simulink model "helix_drone_competition"  (R2022b)
settings: Solver=VariableStepAuto  StartTime=0.0  StopTime=10.0  RelTol=1e-3
settings Model: Creator=gerve  LastModifiedBy=gerve

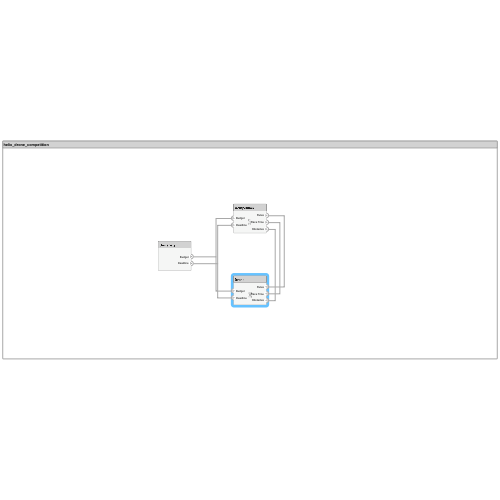
[thumbnail: Simulink's stored preview of the top-level diagram]
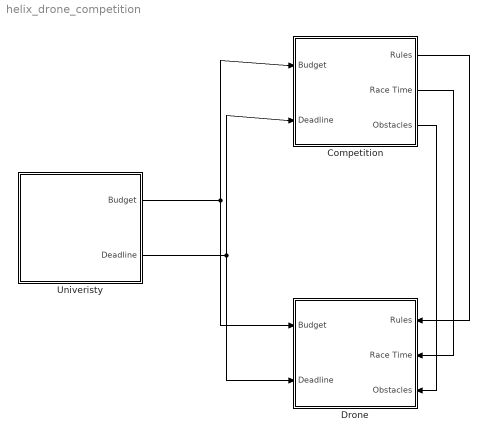
== system helix_drone_competition ==
  Competition : Subsystem
      settings: PortSchema="{\"entries\":[{\"content\":{\"headerSize\":26,\"margin\":15,\"minimumSpacing\":25,\"sides\":[{\"content\":{\"connectorIds\":[\"In1\",\"In2\"]},\"type\":\"ConnectorPlacement.EquallySpacedRectSide\",\"uuid\":\"f32b2b14-41b4-41d2-98c7-b99e10502cf5\"},{\"content\":{\"connectorIds\":[\"Out1\",\"Out2\",\"Out3\"],\"side\":\"RIGHT\"},\"type\":\"ConnectorPlacement.EquallySpacedRectSide\",\"uuid\":\"ebd87c84-7864-4900-8797-b3d9295a8a40\"},{\"content\":{\"connectorIds\":[],\"side\":\"TOP\"},\"type\":\"ConnectorPlacement.EquallySpacedRectSide\",\"uuid\":\"98bce1a8-04c7-44b4-bd36-c653bce1592e\"}]},\"type\":\"ConnectorPlacement.EquallySpacedConnector\",\"uuid\":\"4aeaf037-8c3a-4b17-97e2-80e7a9f8e112\"}],\"packageUris\":[\"http://schema.mathworks.com/mf0/Connector/R2020b\"],\"version\":\"1.0\"}"
  Drone : Subsystem  RequirementInfo="{}  %GIDa_630028c7_c920_43e1_b933_7776371f28a3"
      settings: PortSchema="{\"entries\":[{\"content\":{\"headerSize\":26,\"margin\":15,\"minimumSpacing\":25,\"sides\":[{\"content\":{\"connectorIds\":[\"In4\",\"In5\"]},\"type\":\"ConnectorPlacement.EquallySpacedRectSide\",\"uuid\":\"f32b2b14-41b4-41d2-98c7-b99e10502cf5\"},{\"content\":{\"connectorIds\":[\"In1\",\"In2\",\"In3\"],\"side\":\"RIGHT\"},\"type\":\"ConnectorPlacement.EquallySpacedRectSide\",\"uuid\":\"ebd87c84-7864-4900-8797-b3d9295a8a40\"},{\"content\":{\"connectorIds\":[],\"side\":\"TOP\"},\"type\":\"ConnectorPlacement.EquallySpacedRectSide\",\"uuid\":\"98bce1a8-04c7-44b4-bd36-c653bce1592e\"}]},\"type\":\"ConnectorPlacement.EquallySpacedConnector\",\"uuid\":\"4aeaf037-8c3a-4b17-97e2-80e7a9f8e112\"}],\"packageUris\":[\"http://schema.mathworks.com/mf0/Connector/R2020b\"],\"version\":\"1.0\"}"
  Univeristy : Subsystem
      settings: PortSchema="{\"entries\":[{\"content\":{\"headerSize\":26,\"margin\":15,\"minimumSpacing\":25,\"sides\":[{\"content\":{\"connectorIds\":[]},\"type\":\"ConnectorPlacement.EquallySpacedRectSide\",\"uuid\":\"f32b2b14-41b4-41d2-98c7-b99e10502cf5\"},{\"content\":{\"connectorIds\":[\"Out1\",\"Out2\"],\"side\":\"RIGHT\"},\"type\":\"ConnectorPlacement.EquallySpacedRectSide\",\"uuid\":\"ebd87c84-7864-4900-8797-b3d9295a8a40\"},{\"content\":{\"connectorIds\":[],\"side\":\"TOP\"},\"type\":\"ConnectorPlacement.EquallySpacedRectSide\",\"uuid\":\"98bce1a8-04c7-44b4-bd36-c653bce1592e\"}]},\"type\":\"ConnectorPlacement.EquallySpacedConnector\",\"uuid\":\"4aeaf037-8c3a-4b17-97e2-80e7a9f8e112\"}],\"packageUris\":[\"http://schema.mathworks.com/mf0/Connector/R2020b\"],\"version\":\"1.0\"}"
  wires:
  Univeristy/1(Budget) -> Competition/1(Budget), Drone/4(Budget)
  Univeristy/2(Deadline) -> Competition/2(Deadline), Drone/5(Deadline)
  Competition/1(Rules) -> Drone/1(Rules)
  Competition/2(Race Time) -> Drone/2(Race Time)
  Competition/3(Obstacles) -> Drone/3(Obstacles)

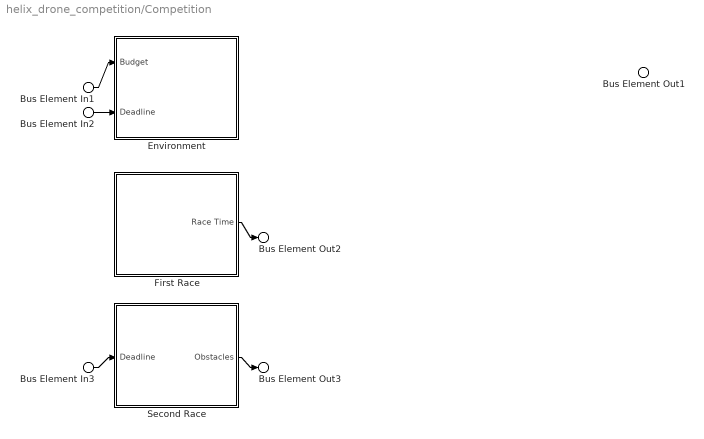
== system helix_drone_competition/Competition ==
  Bus Element In1 : Inport  PortName=Budget
  Bus Element In3 : Inport  PortName=Budget
  Bus Element In2 : Inport  Port=2  PortName=Deadline
  Environment : Subsystem
      settings: PortSchema="{\"entries\":[{\"content\":{\"headerSize\":26,\"margin\":15,\"minimumSpacing\":25,\"sides\":[{\"content\":{\"connectorIds\":[\"In1\",\"In2\"]},\"type\":\"ConnectorPlacement.EquallySpacedRectSide\",\"uuid\":\"f32b2b14-41b4-41d2-98c7-b99e10502cf5\"},{\"content\":{\"connectorIds\":[],\"side\":\"RIGHT\"},\"type\":\"ConnectorPlacement.EquallySpacedRectSide\",\"uuid\":\"ebd87c84-7864-4900-8797-b3d9295a8a40\"},{\"content\":{\"connectorIds\":[],\"side\":\"TOP\"},\"type\":\"ConnectorPlacement.EquallySpacedRectSide\",\"uuid\":\"98bce1a8-04c7-44b4-bd36-c653bce1592e\"}]},\"type\":\"ConnectorPlacement.EquallySpacedConnector\",\"uuid\":\"4aeaf037-8c3a-4b17-97e2-80e7a9f8e112\"}],\"packageUris\":[\"http://schema.mathworks.com/mf0/Connector/R2020b\"],\"version\":\"1.0\"}"
  First Race : Subsystem
      settings: PortSchema="{\"entries\":[{\"content\":{\"headerSize\":26,\"margin\":15,\"minimumSpacing\":25,\"sides\":[{\"content\":{\"connectorIds\":[]},\"type\":\"ConnectorPlacement.EquallySpacedRectSide\",\"uuid\":\"f32b2b14-41b4-41d2-98c7-b99e10502cf5\"},{\"content\":{\"connectorIds\":[\"Out1\"],\"side\":\"RIGHT\"},\"type\":\"ConnectorPlacement.EquallySpacedRectSide\",\"uuid\":\"ebd87c84-7864-4900-8797-b3d9295a8a40\"},{\"content\":{\"connectorIds\":[],\"side\":\"TOP\"},\"type\":\"ConnectorPlacement.EquallySpacedRectSide\",\"uuid\":\"98bce1a8-04c7-44b4-bd36-c653bce1592e\"}]},\"type\":\"ConnectorPlacement.EquallySpacedConnector\",\"uuid\":\"4aeaf037-8c3a-4b17-97e2-80e7a9f8e112\"}],\"packageUris\":[\"http://schema.mathworks.com/mf0/Connector/R2020b\"],\"version\":\"1.0\"}"
  Second Race : Subsystem
      settings: PortSchema="{\"entries\":[{\"content\":{\"headerSize\":26,\"margin\":15,\"minimumSpacing\":25,\"sides\":[{\"content\":{\"connectorIds\":[\"In1\"]},\"type\":\"ConnectorPlacement.EquallySpacedRectSide\",\"uuid\":\"f32b2b14-41b4-41d2-98c7-b99e10502cf5\"},{\"content\":{\"connectorIds\":[\"Out1\"],\"side\":\"RIGHT\"},\"type\":\"ConnectorPlacement.EquallySpacedRectSide\",\"uuid\":\"ebd87c84-7864-4900-8797-b3d9295a8a40\"},{\"content\":{\"connectorIds\":[],\"side\":\"TOP\"},\"type\":\"ConnectorPlacement.EquallySpacedRectSide\",\"uuid\":\"98bce1a8-04c7-44b4-bd36-c653bce1592e\"}]},\"type\":\"ConnectorPlacement.EquallySpacedConnector\",\"uuid\":\"4aeaf037-8c3a-4b17-97e2-80e7a9f8e112\"}],\"packageUris\":[\"http://schema.mathworks.com/mf0/Connector/R2020b\"],\"version\":\"1.0\"}"
  Bus Element Out1 : Outport  PortName=Rules
  Bus Element Out2 : Outport  Port=2  PortName=Race Time
  Bus Element Out3 : Outport  Port=3  PortName=Obstacles
  wires:
  Bus Element In1/1 -> Environment/1(Budget)
  Second Race/1(Obstacles) -> Bus Element Out3/1
  First Race/1(Race Time) -> Bus Element Out2/1
  Bus Element In3/1 -> Second Race/1(Deadline)
  Bus Element In2/1 -> Environment/2(Deadline)

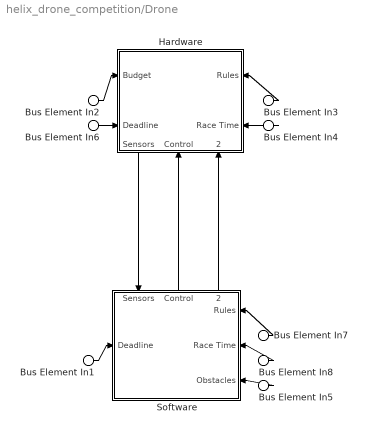
== system helix_drone_competition/Drone ==
  Bus Element In3 : Inport  PortName=Rules
  Bus Element In7 : Inport  PortName=Rules
  Bus Element In4 : Inport  Port=2  PortName=Race Time
  Bus Element In8 : Inport  Port=2  PortName=Race Time
  Bus Element In5 : Inport  Port=3  PortName=Obstacles
  Bus Element In2 : Inport  Port=4  PortName=Budget
  Bus Element In1 : Inport  Port=5  PortName=Deadline
  Bus Element In6 : Inport  Port=5  PortName=Deadline
  Hardware : Subsystem
      settings: PortSchema="{\"entries\":[{\"content\":{\"headerSize\":26,\"margin\":15,\"minimumSpacing\":25,\"sides\":[{\"content\":{\"connectorIds\":[\"In5\",\"In6\"]},\"type\":\"ConnectorPlacement.EquallySpacedRectSide\",\"uuid\":\"f32b2b14-41b4-41d2-98c7-b99e10502cf5\"},{\"content\":{\"connectorIds\":[\"In3\",\"In4\"],\"side\":\"RIGHT\"},\"type\":\"ConnectorPlacement.EquallySpacedRectSide\",\"uuid\":\"ebd87c84-7864-4900-8797-b3d9295a8a40\"},{\"content\":{\"connectorIds\":[],\"side\":\"TOP\"},\"type\":\"ConnectorPlacement.EquallySpacedRectSide\",\"uuid\":\"98bce1a8-04c7-44b4-bd36-c653bce1592e\"},{\"content\":{\"connectorIds\":[\"Out1\",\"In1\",\"In2\"],\"side\":\"BOTTOM\"},\"type\":\"ConnectorPlacement.EquallySpacedRectSide\",\"uuid\":\"b8bbf94b-b15d-45e5-9284-c94e35cda025\"}]},\"type\":\"ConnectorPlacement.EquallySpacedConnector\",\"uuid\":\"4aeaf037-8c3a-4b17-97e2-80e7a9f8e112\"}],\"packageUris\":[\"http://schema.mathworks.com/mf0/Connector/R2020b\"],\"version\":\"1.0\"}"
  Software : Subsystem
      settings: PortSchema="{\"entries\":[{\"content\":{\"headerSize\":26,\"margin\":15,\"minimumSpacing\":25,\"sides\":[{\"content\":{\"connectorIds\":[\"In5\"]},\"type\":\"ConnectorPlacement.EquallySpacedRectSide\",\"uuid\":\"f32b2b14-41b4-41d2-98c7-b99e10502cf5\"},{\"content\":{\"connectorIds\":[\"In2\",\"In3\",\"In4\"],\"side\":\"RIGHT\"},\"type\":\"ConnectorPlacement.EquallySpacedRectSide\",\"uuid\":\"ebd87c84-7864-4900-8797-b3d9295a8a40\"},{\"content\":{\"connectorIds\":[\"In1\",\"Out1\",\"Out2\"],\"side\":\"TOP\"},\"type\":\"ConnectorPlacement.EquallySpacedRectSide\",\"uuid\":\"98bce1a8-04c7-44b4-bd36-c653bce1592e\"},{\"content\":{\"connectorIds\":[],\"side\":\"BOTTOM\"},\"type\":\"ConnectorPlacement.EquallySpacedRectSide\",\"uuid\":\"176a6af5-98df-42e2-83ff-7372f5d8c599\"}]},\"type\":\"ConnectorPlacement.EquallySpacedConnector\",\"uuid\":\"4aeaf037-8c3a-4b17-97e2-80e7a9f8e112\"}],\"packageUris\":[\"http://schema.mathworks.com/mf0/Connector/R2020b\"],\"version\":\"1.0\"}"
  wires:
  Bus Element In2/1 -> Hardware/5(Budget)
  Bus Element In1/1 -> Software/5(Deadline)
  Bus Element In6/1 -> Hardware/6(Deadline)
  Bus Element In3/1 -> Hardware/3(Rules)
  Bus Element In7/1 -> Software/2(Rules)
  Bus Element In4/1 -> Hardware/4(Race Time)
  Bus Element In8/1 -> Software/3(Race Time)
  Bus Element In5/1 -> Software/4(Obstacles)
  Software/2(Instructions) -> Hardware/2(Instructions)
  Hardware/1(Sensors) -> Software/1(Sensors)
  Software/1(Control) -> Hardware/1(Control)

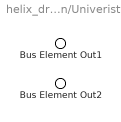
== system helix_drone_competition/Univeristy ==
  Bus Element Out1 : Outport  PortName=Budget
  Bus Element Out2 : Outport  Port=2  PortName=Deadline

== system helix_drone_competition/Competition/Environment ==
  Bus Element In1 : Inport  PortName=Budget
  Bus Element In2 : Inport  Port=2  PortName=Deadline

== system helix_drone_competition/Competition/First Race ==
  Bus Element Out1 : Outport  PortName=Race Time

== system helix_drone_competition/Competition/Second Race ==
  Bus Element In1 : Inport  PortName=Deadline
  Bus Element Out1 : Outport  PortName=Obstacles

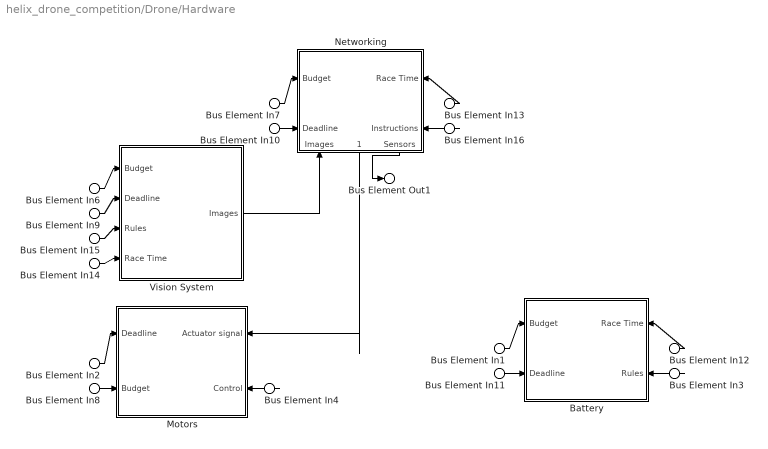
== system helix_drone_competition/Drone/Hardware ==
  Bus Element In4 : Inport  PortName=Control
  Bus Element In16 : Inport  Port=2  PortName=Instructions
  Bus Element In3 : Inport  Port=3  PortName=Rules
  Bus Element In15 : Inport  Port=3  PortName=Rules
  Bus Element In12 : Inport  Port=4  PortName=Race Time
  Bus Element In13 : Inport  Port=4  PortName=Race Time
  Bus Element In14 : Inport  Port=4  PortName=Race Time
  Bus Element In{1,6..8} (4 alike) : Inport  Port=5  PortName=Budget
  Bus Element In{2,9..11} (4 alike) : Inport  Port=6  PortName=Deadline
  Battery : Subsystem
      settings: PortSchema="{\"entries\":[{\"content\":{\"headerSize\":26,\"margin\":15,\"minimumSpacing\":25,\"sides\":[{\"content\":{\"connectorIds\":[\"In3\",\"In4\"]},\"type\":\"ConnectorPlacement.EquallySpacedRectSide\",\"uuid\":\"f32b2b14-41b4-41d2-98c7-b99e10502cf5\"},{\"content\":{\"connectorIds\":[\"In1\",\"In2\"],\"side\":\"RIGHT\"},\"type\":\"ConnectorPlacement.EquallySpacedRectSide\",\"uuid\":\"ebd87c84-7864-4900-8797-b3d9295a8a40\"},{\"content\":{\"connectorIds\":[],\"side\":\"TOP\"},\"type\":\"ConnectorPlacement.EquallySpacedRectSide\",\"uuid\":\"98bce1a8-04c7-44b4-bd36-c653bce1592e\"}]},\"type\":\"ConnectorPlacement.EquallySpacedConnector\",\"uuid\":\"4aeaf037-8c3a-4b17-97e2-80e7a9f8e112\"}],\"packageUris\":[\"http://schema.mathworks.com/mf0/Connector/R2020b\"],\"version\":\"1.0\"}"
  Motors : Subsystem
      settings: PortSchema="{\"entries\":[{\"content\":{\"headerSize\":26,\"margin\":15,\"minimumSpacing\":25,\"sides\":[{\"content\":{\"connectorIds\":[\"In3\",\"In4\"]},\"type\":\"ConnectorPlacement.EquallySpacedRectSide\",\"uuid\":\"f32b2b14-41b4-41d2-98c7-b99e10502cf5\"},{\"content\":{\"connectorIds\":[\"In1\",\"In2\"],\"side\":\"RIGHT\"},\"type\":\"ConnectorPlacement.EquallySpacedRectSide\",\"uuid\":\"ebd87c84-7864-4900-8797-b3d9295a8a40\"},{\"content\":{\"connectorIds\":[],\"side\":\"TOP\"},\"type\":\"ConnectorPlacement.EquallySpacedRectSide\",\"uuid\":\"98bce1a8-04c7-44b4-bd36-c653bce1592e\"}]},\"type\":\"ConnectorPlacement.EquallySpacedConnector\",\"uuid\":\"4aeaf037-8c3a-4b17-97e2-80e7a9f8e112\"}],\"packageUris\":[\"http://schema.mathworks.com/mf0/Connector/R2020b\"],\"version\":\"1.0\"}"
  Networking : Subsystem
      settings: PortSchema="{\"entries\":[{\"content\":{\"headerSize\":26,\"margin\":15,\"minimumSpacing\":25,\"sides\":[{\"content\":{\"connectorIds\":[\"In4\",\"In5\"]},\"type\":\"ConnectorPlacement.EquallySpacedRectSide\",\"uuid\":\"f32b2b14-41b4-41d2-98c7-b99e10502cf5\"},{\"content\":{\"connectorIds\":[\"In2\",\"In3\"],\"side\":\"RIGHT\"},\"type\":\"ConnectorPlacement.EquallySpacedRectSide\",\"uuid\":\"ebd87c84-7864-4900-8797-b3d9295a8a40\"},{\"content\":{\"connectorIds\":[],\"side\":\"TOP\"},\"type\":\"ConnectorPlacement.EquallySpacedRectSide\",\"uuid\":\"98bce1a8-04c7-44b4-bd36-c653bce1592e\"},{\"content\":{\"connectorIds\":[\"In1\",\"Out1\",\"Out2\"],\"side\":\"BOTTOM\"},\"type\":\"ConnectorPlacement.EquallySpacedRectSide\",\"uuid\":\"347c56eb-8d07-4315-bae9-6dad91ea2500\"}]},\"type\":\"ConnectorPlacement.EquallySpacedConnector\",\"uuid\":\"4aeaf037-8c3a-4b17-97e2-80e7a9f8e112\"}],\"packageUris\":[\"http://schema.mathworks.com/mf0/Connector/R2020b\"],\"version\":\"1.0\"}"
  Vision System : Subsystem
      settings: PortSchema="{\"entries\":[{\"content\":{\"headerSize\":26,\"margin\":15,\"minimumSpacing\":25,\"sides\":[{\"content\":{\"connectorIds\":[\"In3\",\"In4\",\"In2\",\"In1\"]},\"type\":\"ConnectorPlacement.EquallySpacedRectSide\",\"uuid\":\"f32b2b14-41b4-41d2-98c7-b99e10502cf5\"},{\"content\":{\"connectorIds\":[\"Out1\"],\"side\":\"RIGHT\"},\"type\":\"ConnectorPlacement.EquallySpacedRectSide\",\"uuid\":\"ebd87c84-7864-4900-8797-b3d9295a8a40\"},{\"content\":{\"connectorIds\":[],\"side\":\"TOP\"},\"type\":\"ConnectorPlacement.EquallySpacedRectSide\",\"uuid\":\"98bce1a8-04c7-44b4-bd36-c653bce1592e\"},{\"content\":{\"connectorIds\":[],\"side\":\"BOTTOM\"},\"type\":\"ConnectorPlacement.EquallySpacedRectSide\",\"uuid\":\"726fdaec-6ead-4202-81de-1add9a01df27\"}]},\"type\":\"ConnectorPlacement.EquallySpacedConnector\",\"uuid\":\"4aeaf037-8c3a-4b17-97e2-80e7a9f8e112\"}],\"packageUris\":[\"http://schema.mathworks.com/mf0/Connector/R2020b\"],\"version\":\"1.0\"}"
  Bus Element Out1 : Outport  PortName=Sensors
  wires:
  Bus Element In9/1 -> Vision System/4(Deadline)
  Bus Element In10/1 -> Networking/5(Deadline)
  Bus Element In11/1 -> Battery/4(Deadline)
  Bus Element In1/1 -> Battery/3(Budget)
  Bus Element In6/1 -> Vision System/3(Budget)
  Bus Element In15/1 -> Vision System/2(Rules)
  Bus Element In14/1 -> Vision System/1(Race Time)
  Bus Element In8/1 -> Motors/4(Budget)
  Bus Element In7/1 -> Networking/4(Budget)
  Vision System/1(Images) -> Networking/1(Images)
  Networking/2(Sensors) -> Bus Element Out1/1
  Networking/1(Actuator signal) -> Motors/1(Actuator signal)
  Bus Element In13/1 -> Networking/2(Race Time)
  Bus Element In12/1 -> Battery/1(Race Time)
  Bus Element In3/1 -> Battery/2(Rules)
  Bus Element In2/1 -> Motors/3(Deadline)
  Bus Element In16/1 -> Networking/3(Instructions)
  Bus Element In4/1 -> Motors/2(Control)

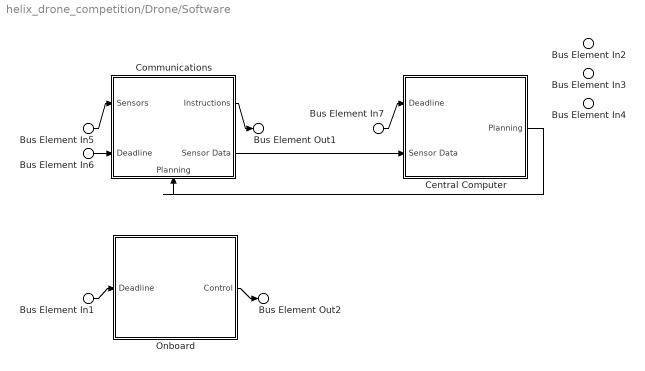
== system helix_drone_competition/Drone/Software ==
  Bus Element In5 : Inport  PortName=Sensors
  Bus Element In2 : Inport  Port=2  PortName=Rules
  Bus Element In3 : Inport  Port=3  PortName=Race Time
  Bus Element In4 : Inport  Port=4  PortName=Obstacles
  Bus Element In1 : Inport  Port=5  PortName=Deadline
  Bus Element In6 : Inport  Port=5  PortName=Deadline
  Bus Element In7 : Inport  Port=5  PortName=Deadline
  Central Computer : Subsystem
      settings: PortSchema="{\"entries\":[{\"content\":{\"headerSize\":26,\"margin\":15,\"minimumSpacing\":25,\"sides\":[{\"content\":{\"connectorIds\":[\"In1\",\"In2\"]},\"type\":\"ConnectorPlacement.EquallySpacedRectSide\",\"uuid\":\"f32b2b14-41b4-41d2-98c7-b99e10502cf5\"},{\"content\":{\"connectorIds\":[\"Out1\"],\"side\":\"RIGHT\"},\"type\":\"ConnectorPlacement.EquallySpacedRectSide\",\"uuid\":\"ebd87c84-7864-4900-8797-b3d9295a8a40\"},{\"content\":{\"connectorIds\":[],\"side\":\"TOP\"},\"type\":\"ConnectorPlacement.EquallySpacedRectSide\",\"uuid\":\"98bce1a8-04c7-44b4-bd36-c653bce1592e\"}]},\"type\":\"ConnectorPlacement.EquallySpacedConnector\",\"uuid\":\"4aeaf037-8c3a-4b17-97e2-80e7a9f8e112\"}],\"packageUris\":[\"http://schema.mathworks.com/mf0/Connector/R2020b\"],\"version\":\"1.0\"}"
  Communications : Subsystem
      settings: PortSchema="{\"entries\":[{\"content\":{\"headerSize\":26,\"margin\":15,\"minimumSpacing\":25,\"sides\":[{\"content\":{\"connectorIds\":[\"In2\",\"In3\"]},\"type\":\"ConnectorPlacement.EquallySpacedRectSide\",\"uuid\":\"f32b2b14-41b4-41d2-98c7-b99e10502cf5\"},{\"content\":{\"connectorIds\":[\"Out1\",\"Out2\"],\"side\":\"RIGHT\"},\"type\":\"ConnectorPlacement.EquallySpacedRectSide\",\"uuid\":\"ebd87c84-7864-4900-8797-b3d9295a8a40\"},{\"content\":{\"connectorIds\":[],\"side\":\"TOP\"},\"type\":\"ConnectorPlacement.EquallySpacedRectSide\",\"uuid\":\"98bce1a8-04c7-44b4-bd36-c653bce1592e\"},{\"content\":{\"connectorIds\":[\"In1\"],\"side\":\"BOTTOM\"},\"type\":\"ConnectorPlacement.EquallySpacedRectSide\",\"uuid\":\"336834bf-44bd-4552-b40f-18addbb842af\"}]},\"type\":\"ConnectorPlacement.EquallySpacedConnector\",\"uuid\":\"4aeaf037-8c3a-4b17-97e2-80e7a9f8e112\"}],\"packageUris\":[\"http://schema.mathworks.com/mf0/Connector/R2020b\"],\"version\":\"1.0\"}"
  Onboard : Subsystem
      settings: PortSchema="{\"entries\":[{\"content\":{\"headerSize\":26,\"margin\":15,\"minimumSpacing\":25,\"sides\":[{\"content\":{\"connectorIds\":[\"In1\"]},\"type\":\"ConnectorPlacement.EquallySpacedRectSide\",\"uuid\":\"f32b2b14-41b4-41d2-98c7-b99e10502cf5\"},{\"content\":{\"connectorIds\":[\"Out1\"],\"side\":\"RIGHT\"},\"type\":\"ConnectorPlacement.EquallySpacedRectSide\",\"uuid\":\"ebd87c84-7864-4900-8797-b3d9295a8a40\"},{\"content\":{\"connectorIds\":[],\"side\":\"TOP\"},\"type\":\"ConnectorPlacement.EquallySpacedRectSide\",\"uuid\":\"98bce1a8-04c7-44b4-bd36-c653bce1592e\"}]},\"type\":\"ConnectorPlacement.EquallySpacedConnector\",\"uuid\":\"4aeaf037-8c3a-4b17-97e2-80e7a9f8e112\"}],\"packageUris\":[\"http://schema.mathworks.com/mf0/Connector/R2020b\"],\"version\":\"1.0\"}"
  Bus Element Out2 : Outport  PortName=Control
  Bus Element Out1 : Outport  Port=2  PortName=Instructions
  wires:
  Bus Element In1/1 -> Onboard/1(Deadline)
  Bus Element In6/1 -> Communications/3(Deadline)
  Bus Element In5/1 -> Communications/2(Sensors)
  Communications/2(Sensor Data) -> Central Computer/2(Sensor Data)
  Communications/1(Instructions) -> Bus Element Out1/1
  Bus Element In7/1 -> Central Computer/1(Deadline)
  Onboard/1(Control) -> Bus Element Out2/1
  Central Computer/1(Planning) -> Communications/1(Planning)

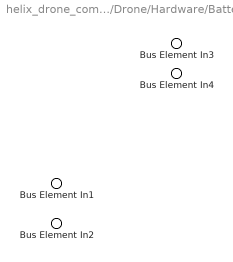
== system helix_drone_competition/Drone/Hardware/Battery ==
  Bus Element In3 : Inport  PortName=Race Time
  Bus Element In4 : Inport  Port=2  PortName=Rules
  Bus Element In1 : Inport  Port=3  PortName=Budget
  Bus Element In2 : Inport  Port=4  PortName=Deadline

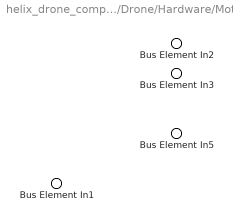
== system helix_drone_competition/Drone/Hardware/Motors ==
  Bus Element In5 : Inport  PortName=Actuator signal
  Bus Element In3 : Inport  Port=2  PortName=Control
  Bus Element In2 : Inport  Port=3  PortName=Deadline
  Bus Element In1 : Inport  Port=4  PortName=Budget

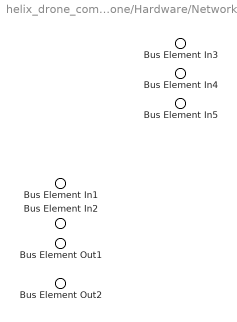
== system helix_drone_competition/Drone/Hardware/Networking ==
  Bus Element In5 : Inport  PortName=Images
  Bus Element In3 : Inport  Port=2  PortName=Race Time
  Bus Element In4 : Inport  Port=3  PortName=Instructions
  Bus Element In1 : Inport  Port=4  PortName=Budget
  Bus Element In2 : Inport  Port=5  PortName=Deadline
  Bus Element Out1 : Outport  PortName=Actuator signal
  Bus Element Out2 : Outport  Port=2  PortName=Sensors

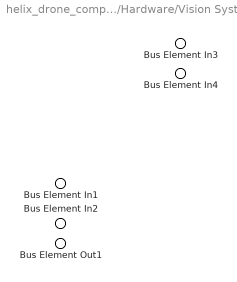
== system helix_drone_competition/Drone/Hardware/Vision System ==
  Bus Element In3 : Inport  PortName=Race Time
  Bus Element In4 : Inport  Port=2  PortName=Rules
  Bus Element In1 : Inport  Port=3  PortName=Budget
  Bus Element In2 : Inport  Port=4  PortName=Deadline
  Bus Element Out1 : Outport  PortName=Images

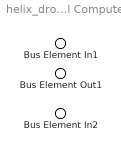
== system helix_drone_competition/Drone/Software/Central Computer ==
  Bus Element In1 : Inport  PortName=Deadline
  Bus Element In2 : Inport  Port=2  PortName=Sensor Data
  Bus Element Out1 : Outport  PortName=Planning

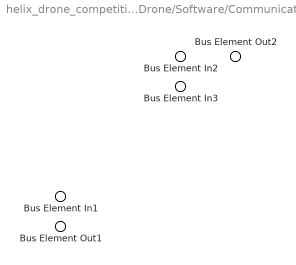
== system helix_drone_competition/Drone/Software/Communications ==
  Bus Element In3 : Inport  PortName=Planning
  Bus Element In2 : Inport  Port=2  PortName=Sensors
  Bus Element In1 : Inport  Port=3  PortName=Deadline
  Bus Element Out2 : Outport  PortName=Instructions
  Bus Element Out1 : Outport  Port=2  PortName=Sensor Data

== system helix_drone_competition/Drone/Software/Onboard ==
  Bus Element In1 : Inport  PortName=Deadline
  Bus Element Out1 : Outport  PortName=Control
